simulink model "PMSM_Motor"  (R2023a)
settings: Solver=ode45  StartTime=0.0  StopTime=0.1  MaxStep=1e-4  RelTol=1e-4  AbsTol=1e-4  EnableMultiTasking=on
libraries: spsControlledVoltageSourceLib x3, spsCurrentMeasurementLib x3, slpidlib x2, spsPermanentMagnetSynchronousMachineLib x1, canoelib x1, sps_lib x1
settings Model: Creator=user  LastModifiedBy=hatep
settings SolverCC: AutoScaleAbsTol=off  AlgebraicLoopSolver=TrustRegion
settings DataIOCC: LimitDataPoints=on  SaveFormat=Array  ReturnWorkspaceOutputs=off
settings OptimizationCC: LifeSpan=inf
settings DebuggingCC: SolverPrmCheckMsg=warning  UnconnectedInputMsg=warning  UnconnectedOutputMsg=warning  UnconnectedLineMsg=warning  SFUnexpectedBacktrackingDiag=warning  SFNoUnconditionalDefaultTransitionDiag=warning  SFExecutionAtInitializationDiag=none  ArithmeticOperatorsInVariantConditions=warning
settings HardwareCC: ProdBitPerPointer=32  ProdBitPerSizeT=32  ProdBitPerPtrDiffT=32  ProdLargestAtomicFloat=None  ProdIntDivRoundTo=Undefined  ProdEndianess=Unspecified  ProdWordSize=32  ProdHWDeviceType=32-bit Generic
settings ModelReferenceCC: PropagateSignalLabelsOutOfModel=off
settings SFSimCC: SimUseLocalCustomCode=off  CustomCodeUndefinedFunction=UseInterfaceOnly
settings RTWCC: RTWUseLocalCustomCode=off
settings CodeAppCC: StateflowObjectComments=on
settings GRTTargetCC: TargetLangStandard=C89/C90 (ANSI)
settings ConfigComp: CovMetricSettings=dw  CovSaveCumulativeToWorkspaceVar=on  CovSaveSingleToWorkspaceVar=on  CovExternalEMLEnable=off  CovSFcnEnable=off
settings SimscapeCC: SimscapeNormalizeSystem=off

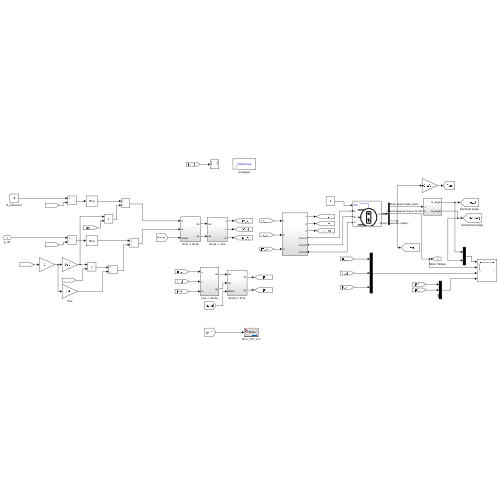
[thumbnail: Simulink's stored preview of the top-level diagram]
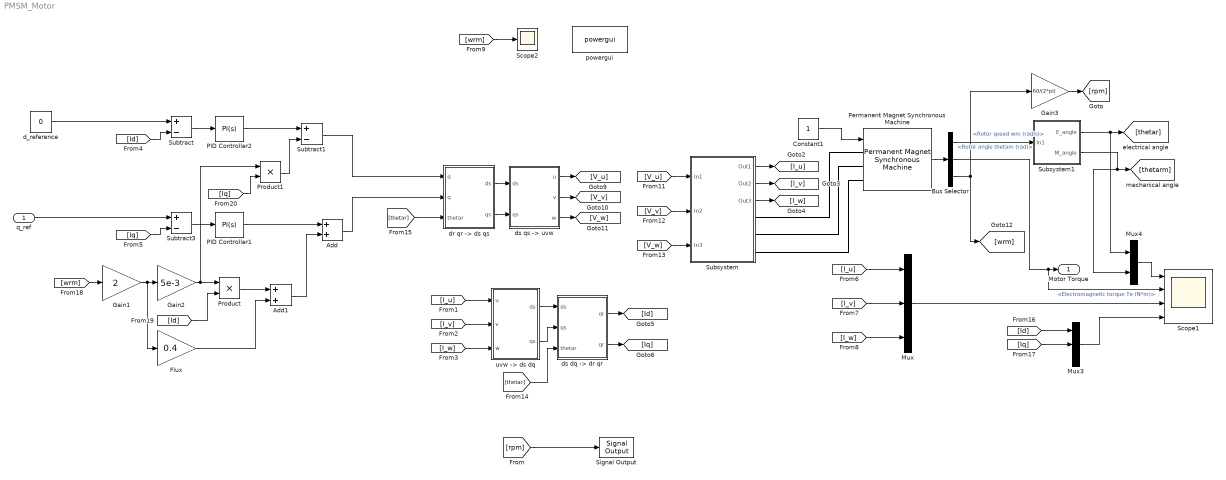
== system PMSM_Motor ==
  q_ref : Inport
  Add : Sum
  Add1 : Sum
  Bus Selector : BusSelector  OutputSignals=Rotor angle thetam (rad),Electromagnetic torque Te (N*m),Rotor speed wm (rad/s)
  Constant1 : Constant
  Flux : Gain  Gain=0.4
  Gain1 : Gain  Gain=2
  Gain2 : Gain  Gain=5e-3
  Gain3 : Gain  Gain=60/(2*pi)
  Mux : Mux  Inputs=3
  Mux3 : Mux  Inputs=3
  Mux4 : Mux  Inputs=2
  PID Controller1 : slpidlib/PID Controller  Controller=PI  Form=Parallel  TimeDomain=Continuous-time  UseExternalTs=off  SampleTime=-1  IntegratorMethod=Forward Euler  FilterMethod=Forward Euler  ControllerParametersSource=internal  P=0.005*500*2*pi  I=0.5*500*2*pi  UseKiTs=off  D=0  N=100  UseFilter=on  TunerSelectOption=Transfer Function Based (PID Tuner App)  InitialConditionSource=internal  InitialConditionForIntegrator=0  InitialConditionForFilter=0  DifferentiatorICPrevScaledInput=0  ExternalReset=none  TrackingMode=off  Kt=1  LimitOutput=off  SatLimitsSource=internal  UpperSaturationLimit=inf  LowerSaturationLimit=-inf  LinearizeAsGain=on  AntiWindupMode=none  Kb=1  LimitIntegrator=off  UpperIntegratorSaturationLimit=inf  LowerIntegratorSaturationLimit=-inf  POutMin=[]  POutMax=[]  IOutMin=[]  IOutMax=[]  DOutMin=[]  DOutMax=[]  NOutMin=[]  NOutMax=[]  SumOutMin=[]  SumOutMax=[]  SaturationOutMin=[]  SaturationOutMax=[]  PParamMin=[]  PParamMax=[]  IParamMin=[]  IParamMax=[]  DParamMin=[]  DParamMax=[]  NParamMin=[]  NParamMax=[]  KbParamMin=[]  KbParamMax=[]  KtParamMin=[]  KtParamMax=[]  KbOutMin=[]  KbOutMax=[]  KtOutMin=[]  KtOutMax=[]  IntegratorOutMin=[]  IntegratorOutMax=[]  FilterOutMin=[]  FilterOutMax=[]  SumI1OutMin=[]  SumI1OutMax=[]  SumI2OutMin=[]  SumI2OutMax=[]  SumI3OutMin=[]  SumI3OutMax=[]  SumI4OutMin=[]  SumI4OutMax=[]  SumDOutMin=[]  SumDOutMax=[]  DifferentiatorOutMin=[]  DifferentiatorOutMax=[]  FilterDiffOutCoefMin=[]  FilterDiffOutCoefMax=[]  ReciprocalOutMin=[]  ReciprocalOutMax=[]  SumDenOutMin=[]  SumDenOutMax=[]  SumNumOutMin=[]  SumNumOutMax=[]  DivideOutMin=[]  DivideOutMax=[]  UdiffTsProdOutMin=[]  UdiffTsProdOutMax=[]  NTsProdOutMin=[]  NTsProdOutMax=[]  UintegralTsProdOutMin=[]  UintegralTsProdOutMax=[]  UngainTsProdOutMin=[]  UngainTsProdOutMax=[]  ClampingZeroOutDataTypeStr=Inherit: Inherit via back propagation  ClampingZeroOutMin=[]  ClampingZeroOutMax=[]  FilterDenConstantOutDataTypeStr=Inherit: Inherit via back propagation  FilterDenConstantOutMin=[]  FilterDenConstantOutMax=[]  PCopyOutDataTypeStr=Inherit: Inherit via back propagation  PCopyOutMin=[]  PCopyOutMax=[]  NCopyOutDataTypeStr=Inherit: Inherit via back propagation  NCopyOutMin=[]  NCopyOutMax=[]  IntegratorContinuousStateAttributes=''  IntegratorStateMustResolveToSignalObject=off  IntegratorRTWStateStorageClass=Auto  FilterContinuousStateAttributes=''  FilterStateMustResolveToSignalObject=off  FilterRTWStateStorageClass=Auto  ParallelPVariant=InternalParameters  IdealPVariant=Disabled  IVariant=InternalParameters  DVariant=Disabled  IntegratorVariant=Continuous  SatVariant=Disabled  AWVariant=Passthrough  PCopyVariant=Disabled  TRVariant=Disabled  FdbkBlocksVariant=Forward  IdealPFdbkVariant=Disabled  SatFdbkVariant=Disabled  DerivativeFilterVariant=Disabled  NVariant=Disabled  NCopyVariant=Disabled_SignalSpec  FilterICVariant=Disabled  IntegratorICVariant=InternalICs  ExternalResetVariant=Disabled  TRSumVariant=Passthrough  SumFdbkVariant=Disabled  SumVariant=Sum_PI  TsampFilterVariant=InternalTs  TsampNgainVariant=Passthrough  TsampIntegralVariant=Disabled_SignalSpec  ExternalSaturationOutDataTypeStr=Inherit: Same as second input
  PID Controller2 : slpidlib/PID Controller  Controller=PI  Form=Parallel  TimeDomain=Continuous-time  UseExternalTs=off  SampleTime=-1  IntegratorMethod=Forward Euler  FilterMethod=Forward Euler  ControllerParametersSource=internal  P=0.005*500*2*pi  I=0.5*500*2*pi  UseKiTs=off  D=0  N=100  UseFilter=on  TunerSelectOption=Transfer Function Based (PID Tuner App)  InitialConditionSource=internal  InitialConditionForIntegrator=0  InitialConditionForFilter=0  DifferentiatorICPrevScaledInput=0  ExternalReset=none  TrackingMode=off  Kt=1  LimitOutput=off  SatLimitsSource=internal  UpperSaturationLimit=inf  LowerSaturationLimit=-inf  LinearizeAsGain=on  AntiWindupMode=none  Kb=1  LimitIntegrator=off  UpperIntegratorSaturationLimit=inf  LowerIntegratorSaturationLimit=-inf  POutMin=[]  POutMax=[]  IOutMin=[]  IOutMax=[]  DOutMin=[]  DOutMax=[]  NOutMin=[]  NOutMax=[]  SumOutMin=[]  SumOutMax=[]  SaturationOutMin=[]  SaturationOutMax=[]  PParamMin=[]  PParamMax=[]  IParamMin=[]  IParamMax=[]  DParamMin=[]  DParamMax=[]  NParamMin=[]  NParamMax=[]  KbParamMin=[]  KbParamMax=[]  KtParamMin=[]  KtParamMax=[]  KbOutMin=[]  KbOutMax=[]  KtOutMin=[]  KtOutMax=[]  IntegratorOutMin=[]  IntegratorOutMax=[]  FilterOutMin=[]  FilterOutMax=[]  SumI1OutMin=[]  SumI1OutMax=[]  SumI2OutMin=[]  SumI2OutMax=[]  SumI3OutMin=[]  SumI3OutMax=[]  SumI4OutMin=[]  SumI4OutMax=[]  SumDOutMin=[]  SumDOutMax=[]  DifferentiatorOutMin=[]  DifferentiatorOutMax=[]  FilterDiffOutCoefMin=[]  FilterDiffOutCoefMax=[]  ReciprocalOutMin=[]  ReciprocalOutMax=[]  SumDenOutMin=[]  SumDenOutMax=[]  SumNumOutMin=[]  SumNumOutMax=[]  DivideOutMin=[]  DivideOutMax=[]  UdiffTsProdOutMin=[]  UdiffTsProdOutMax=[]  NTsProdOutMin=[]  NTsProdOutMax=[]  UintegralTsProdOutMin=[]  UintegralTsProdOutMax=[]  UngainTsProdOutMin=[]  UngainTsProdOutMax=[]  ClampingZeroOutDataTypeStr=Inherit: Inherit via back propagation  ClampingZeroOutMin=[]  ClampingZeroOutMax=[]  FilterDenConstantOutDataTypeStr=Inherit: Inherit via back propagation  FilterDenConstantOutMin=[]  FilterDenConstantOutMax=[]  PCopyOutDataTypeStr=Inherit: Inherit via back propagation  PCopyOutMin=[]  PCopyOutMax=[]  NCopyOutDataTypeStr=Inherit: Inherit via back propagation  NCopyOutMin=[]  NCopyOutMax=[]  IntegratorContinuousStateAttributes=''  IntegratorStateMustResolveToSignalObject=off  IntegratorRTWStateStorageClass=Auto  FilterContinuousStateAttributes=''  FilterStateMustResolveToSignalObject=off  FilterRTWStateStorageClass=Auto  ParallelPVariant=InternalParameters  IdealPVariant=Disabled  IVariant=InternalParameters  DVariant=Disabled  IntegratorVariant=Continuous  SatVariant=Disabled  AWVariant=Passthrough  PCopyVariant=Disabled  TRVariant=Disabled  FdbkBlocksVariant=Forward  IdealPFdbkVariant=Disabled  SatFdbkVariant=Disabled  DerivativeFilterVariant=Disabled  NVariant=Disabled  NCopyVariant=Disabled_SignalSpec  FilterICVariant=Disabled  IntegratorICVariant=InternalICs  ExternalResetVariant=Disabled  TRSumVariant=Passthrough  SumFdbkVariant=Disabled  SumVariant=Sum_PI  TsampFilterVariant=InternalTs  TsampNgainVariant=Passthrough  TsampIntegralVariant=Disabled_SignalSpec  ExternalSaturationOutDataTypeStr=Inherit: Same as second input
  Permanent Magnet Synchronous Machine : spsPermanentMagnetSynchronousMachineLib/Permanent Magnet Synchronous Machine  NbPhases=3  FluxDistribution=Sinusoidal  RotorType=Round  MechanicalLoad=Torque Tm  PresetModel=No  ShowDetailedParameters=on  MeasurementBus=off  Resistance=0.5  Inductance=8.5e-3  dqInductances=[8.5e-3,8.5e-3]  La=0.005  MachineConstant=Flux linkage established by magnets (V.s)  Flux=0.4  VoltageCst=145.1039  TorqueCst=1.2  Flat=120  Mechanical=[0.003 0.004 2 0]  PolePairs=2  InitialConditions=[0,0, 0,0]  InitialConditions5ph=[0 0 0 0 0 0]  RefAngle=Aligned with phase A axis (original Park)  IterativeDiscreteModel=Trapezoidal non iterative  TsBlock=-1  TsPowergui=0
  Product : Product
  Product1 : Product
  Scope1 : Scope  NumInputPorts=4
  Scope2 : Scope
  Signal Output : canoelib/CANoe I//O/Signal Output  dbName=MBD  nodeName=MainCtr  msgName=Ctr  sigName=Main_RW_rpm  rawValue=Raw value  dataType=Default  dataTypeDB=uint16  hasEncoding=off
      settings: AttributesFormatString=%<sigName>  SourceProductName=Vector CANoe
  Subsystem : Subsystem
  Subsystem1 : Subsystem
  Subtract : Sum  Inputs=+-
  Subtract1 : Sum  Inputs=+-
  Subtract3 : Sum  Inputs=+-
  d_reference : Constant  Value=0
  "dr qr -> ds qs" : Subsystem
  "ds dq -> dr qr" : Subsystem
  "ds qs -> uvw" : Subsystem
  powergui : sps_lib/powergui  Priority=1  SimulationMode=Continuous  SampleTime=50e-6  frequency=60  Iterations=50  frequencyindice=0  Pbase=100e6  ErrMax=1e-4  UnitsV=kV  UnitsW=MW  buscounter=0  FunctionMessages=off  echomessages=off  EnableUseOfTLC=off  CurrentSourceSwitches=off  DisableSnubberDevices=off  DisableRonSwitches=off  DisableVfSwitches=off  DisplayEquations=off  AutomaticDiscreteSolvers=off  SolverType=Tustin/Backward Euler (TBE)  Interpol=off  ExternalGateDelay=off  methode=off  Ts=100  x0status=blocks  SPID=on  SwTol=0  HookPort=off  NonlinearTolerance=1e-4  nMaxIteration=100  ContinueOnMaxIteration=off  RestoreLinks=warning  ResistiveCurrentMeasurement=off  Frange=[0:2:500]  Ylog=off  Xlog=on  ShowGrid=off  save=off  variable=ZData  structure=0  ZoomFFT=off  StartTime=0.0  cycles=1  DisplayStyle=1  fundamental=60  FreqAxis=off  MaxFrequency=1000  frequencyindicesteady=1  RmsSteady=1  display=off
  "uvw -> ds dq" : Subsystem
  Motor Torque : Outport
  wires:
  Subtract/1 -> PID Controller2/1
  Permanent Magnet Synchronous Machine/1 -> Bus Selector/1
  Mux/1 -> Scope1/3
  Bus Selector/2 -> Scope1/2, Motor Torque/1  "<Electromagnetic torque Te (N*m)>"
  Subtract3/1 -> PID Controller1/1
  Subsystem/1(Out1) -> [I_u]
  Subsystem/2(Out2) -> [I_v]
  Subsystem/3(Out3) -> [I_w]
  [Id] -> Subtract/2
  [Iq] -> Subtract3/2
  [I_u] -> Mux/1
  [I_v] -> Mux/2
  [I_w] -> Mux/3
  Mux3/1 -> Scope1/4
  [Id] -> Mux3/1
  [Iq] -> Mux3/2
  "dr qr -> ds qs"/1(ds) -> "ds qs -> uvw"/1(ds)
  "dr qr -> ds qs"/2(qs) -> "ds qs -> uvw"/2(qs)
  "ds qs -> uvw"/1(u) -> [V_u]
  "ds qs -> uvw"/2(v) -> [V_v]
  "ds qs -> uvw"/3(w) -> [V_w]
  [I_u] -> "uvw -> ds dq"/1(u)
  [I_v] -> "uvw -> ds dq"/2(v)
  [I_w] -> "uvw -> ds dq"/3(w)
  [V_w] -> Subsystem/3(In3)
  [V_v] -> Subsystem/2(In2)
  [V_u] -> Subsystem/1(In1)
  Bus Selector/3 -> [wrm], Gain3/1  "<Rotor speed wm (rad/s)>"
  "uvw -> ds dq"/1(ds) -> "ds dq -> dr qr"/1(ds)
  "uvw -> ds dq"/2(qs) -> "ds dq -> dr qr"/2(qs)
  "ds dq -> dr qr"/1(dr) -> [Id]
  "ds dq -> dr qr"/2(qr) -> [Iq]
  [thetar] -> "ds dq -> dr qr"/3(thetar)
  Add/1 -> "dr qr -> ds qs"/2(q)
  Subtract1/1 -> "dr qr -> ds qs"/1(d)
  [thetar] -> "dr qr -> ds qs"/3(thetar)
  PID Controller1/1 -> Add/1
  [wrm] -> Gain1/1
  Gain1/1 -> Flux/1, Gain2/1
  Gain2/1 -> Product1/1, Product/1
  [Id] -> Product/2
  Product/1 -> Add1/1
  Flux/1 -> Add1/2
  PID Controller2/1 -> Subtract1/1
  [Iq] -> Product1/2
  Product1/1 -> Subtract1/2
  Add1/1 -> Add/2
  Mux4/1 -> Scope1/1
  Subsystem1/1(E_angle) -> Mux4/1, [thetar]
  Subsystem1/2(M_angle) -> Mux4/2, [thetarm]
  Bus Selector/1 -> Subsystem1/1(In1)  "<Rotor angle thetam (rad)>"
  Gain3/1 -> [rpm]
  d_reference/1 -> Subtract/1
  Constant1/1 -> Permanent Magnet Synchronous Machine/1
  [wrm] -> Scope2/1
  [rpm] -> Signal Output/1
  q_ref/1 -> Subtract3/1
  connections:
  Subsystem/RConn1 -- Permanent Magnet Synchronous Machine/LConn1
  Subsystem/RConn2 -- Permanent Magnet Synchronous Machine/LConn2
  Subsystem/RConn3 -- Permanent Magnet Synchronous Machine/LConn3

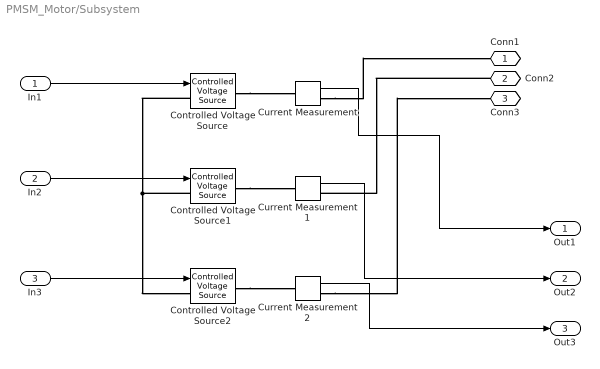
== system PMSM_Motor/Subsystem ==
  In1 : Inport
  In2 : Inport  Port=2
  In3 : Inport  Port=3
  Controlled Voltage Source : spsControlledVoltageSourceLib/Controlled Voltage Source  Initialize=on  Source_Type=AC  Amplitude=0  Phase=0  Frequency=0  Measurements=None
  Controlled Voltage Source1 : spsControlledVoltageSourceLib/Controlled Voltage Source  Initialize=on  Source_Type=AC  Amplitude=0  Phase=0  Frequency=0  Measurements=None
  Controlled Voltage Source2 : spsControlledVoltageSourceLib/Controlled Voltage Source  Initialize=on  Source_Type=AC  Amplitude=0  Phase=0  Frequency=0  Measurements=None
  Current Measurement : spsCurrentMeasurementLib/Current Measurement  PhasorSimulation=off  OutputType=Complex  PSBequivalent=0
  Current Measurement1 : spsCurrentMeasurementLib/Current Measurement  PhasorSimulation=off  OutputType=Complex  PSBequivalent=0
  Current Measurement2 : spsCurrentMeasurementLib/Current Measurement  PhasorSimulation=off  OutputType=Complex  PSBequivalent=0
  Conn1 : PMIOPort  Side=Right
  Conn2 : PMIOPort  Port=2  Side=Right
  Conn3 : PMIOPort  Port=3  Side=Right
  Out1 : Outport
  Out2 : Outport  Port=2
  Out3 : Outport  Port=3
  wires:
  Current Measurement1/1 -> Out2/1
  In3/1 -> Controlled Voltage Source2/1
  In2/1 -> Controlled Voltage Source1/1
  In1/1 -> Controlled Voltage Source/1
  Current Measurement2/1 -> Out3/1
  Current Measurement/1 -> Out1/1
  connections:
  Current Measurement/RConn1 -- Conn1/RConn1
  Controlled Voltage Source/LConn1 -- Controlled Voltage Source1/LConn1 -- Controlled Voltage Source2/LConn1
  Controlled Voltage Source/RConn1 -- Current Measurement/LConn1
  Conn2/RConn1 -- Current Measurement1/RConn1
  Current Measurement2/RConn1 -- Conn3/RConn1
  Controlled Voltage Source1/RConn1 -- Current Measurement1/LConn1
  Controlled Voltage Source2/RConn1 -- Current Measurement2/LConn1

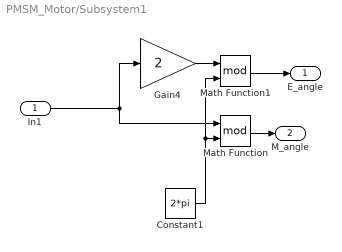
== system PMSM_Motor/Subsystem1 ==
  In1 : Inport
  Constant1 : Constant  Value=2*pi
  Gain4 : Gain  Gain=2
  Math Function : Math  Operator=mod  SignedPower=on
  Math Function1 : Math  Operator=mod  SignedPower=on
  E_angle : Outport
  M_angle : Outport  Port=2
  wires:
  In1/1 -> Gain4/1, Math Function/1
  Constant1/1 -> Math Function1/2, Math Function/2
  Math Function/1 -> M_angle/1
  Gain4/1 -> Math Function1/1
  Math Function1/1 -> E_angle/1

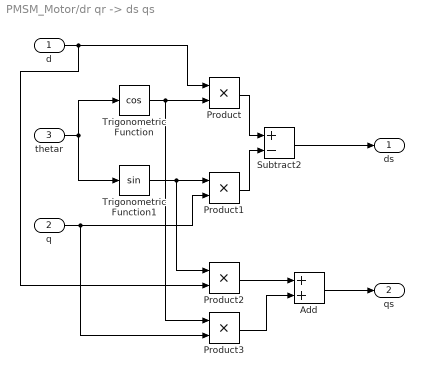
== system PMSM_Motor/dr qr -> ds qs ==
  d : Inport
  q : Inport  Port=2
  thetar : Inport  Port=3
  Add : Sum
  Product{,1..3} (4 alike) : Product
  Subtract2 : Sum  Inputs=+-
  Trigonometric Function : Trigonometry  Operator=cos
  Trigonometric Function1 : Trigonometry
  ds : Outport
  qs : Outport  Port=2
  wires:
  Product3/1 -> Add/2
  Product2/1 -> Add/1
  d/1 -> Product2/2, Product/1
  Add/1 -> qs/1
  Subtract2/1 -> ds/1
  Product1/1 -> Subtract2/2
  Product/1 -> Subtract2/1
  q/1 -> Product1/2, Product3/2
  Trigonometric Function1/1 -> Product1/1, Product2/1
  Trigonometric Function/1 -> Product/2, Product3/1
  thetar/1 -> Trigonometric Function1/1, Trigonometric Function/1

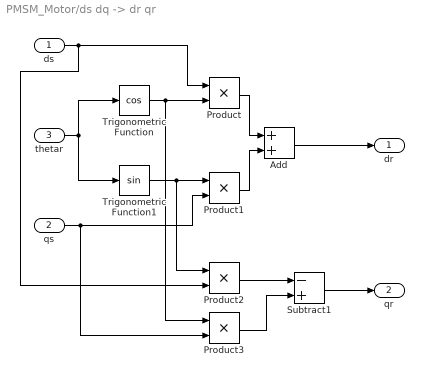
== system PMSM_Motor/ds dq -> dr qr ==
  ds : Inport
  qs : Inport  Port=2
  thetar : Inport  Port=3
  Add : Sum
  Product{,1..3} (4 alike) : Product
  Subtract1 : Sum  Inputs=-+
  Trigonometric Function : Trigonometry  Operator=cos
  Trigonometric Function1 : Trigonometry
  dr : Outport
  qr : Outport  Port=2
  wires:
  thetar/1 -> Trigonometric Function/1, Trigonometric Function1/1
  Trigonometric Function/1 -> Product3/1, Product/2
  Trigonometric Function1/1 -> Product2/1, Product1/1
  qs/1 -> Product3/2, Product1/2
  Product/1 -> Add/1
  Product1/1 -> Add/2
  Add/1 -> dr/1
  Subtract1/1 -> qr/1
  ds/1 -> Product/1, Product2/2
  Product2/1 -> Subtract1/1
  Product3/1 -> Subtract1/2

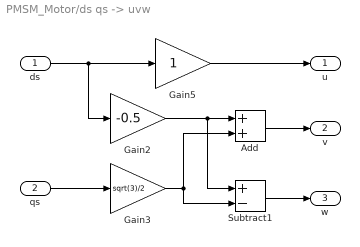
== system PMSM_Motor/ds qs -> uvw ==
  ds : Inport
  qs : Inport  Port=2
  Add : Sum
  Gain2 : Gain  Gain=-0.5
  Gain3 : Gain  Gain=sqrt(3)/2
  Gain5 : Gain
  Subtract1 : Sum  Inputs=+-
  u : Outport
  v : Outport  Port=2
  w : Outport  Port=3
  wires:
  ds/1 -> Gain2/1, Gain5/1
  Gain3/1 -> Subtract1/2, Add/2
  Gain2/1 -> Subtract1/1, Add/1
  Add/1 -> v/1
  Subtract1/1 -> w/1
  qs/1 -> Gain3/1
  Gain5/1 -> u/1

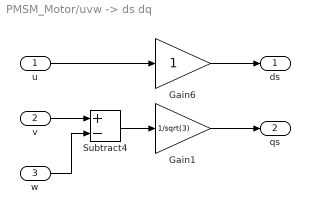
== system PMSM_Motor/uvw -> ds dq ==
  u : Inport
  v : Inport  Port=2
  w : Inport  Port=3
  Gain1 : Gain  Gain=1/sqrt(3)
  Gain6 : Gain
  Subtract4 : Sum  Inputs=+-
  ds : Outport
  qs : Outport  Port=2
  wires:
  v/1 -> Subtract4/1
  u/1 -> Gain6/1
  w/1 -> Subtract4/2
  Gain1/1 -> qs/1
  Subtract4/1 -> Gain1/1
  Gain6/1 -> ds/1
